simulink model "virtual_hopper_feedback_simplified"  (R2018b)
settings: Solver=ode4  StartTime=0  StopTime=10  FixedStep=0.0005  RelTol=1e-7  AbsTol=1e-9  EnableMultiTasking=on
settings Model: Creator=Laksh  LastModifiedBy=Ko
settings SolverCC: AutoScaleAbsTol=off  MaxConsecutiveMinStep=10  AlgebraicLoopSolver=LineSearch
settings DataIOCC: SaveFormat=StructureWithTime  SignalLogging=off  ReturnWorkspaceOutputs=on
settings OptimizationCC: LifeSpan=inf
settings DebuggingCC: ReadBeforeWriteMsg=DisableAll  WriteAfterWriteMsg=DisableAll  WriteAfterReadMsg=DisableAll  AlgebraicLoopMsg=none  MultiTaskDSMMsg=none  SFUnexpectedBacktrackingDiag=warning  SFNoUnconditionalDefaultTransitionDiag=warning  SFExecutionAtInitializationDiag=none
settings ModelReferenceCC: UpdateModelReferenceTargets=IfOutOfDate  ModelReferenceMinAlgLoopOccurrences=on
settings SFSimCC: SFSimEcho=off  SimUseLocalCustomCode=off
settings RTWCC: RTWUseLocalCustomCode=off
settings CodeAppCC: StateflowObjectComments=on
settings GRTTargetCC: TargetLangStandard=C89/C90 (ANSI)  GeneratePreprocessorConditionals=Disable all
settings ConfigComp: CovMetricSettings=dw  CovHtmlReporting=on  CovSaveCumulativeToWorkspaceVar=on  CovSaveSingleToWorkspaceVar=on  CovExternalEMLEnable=off

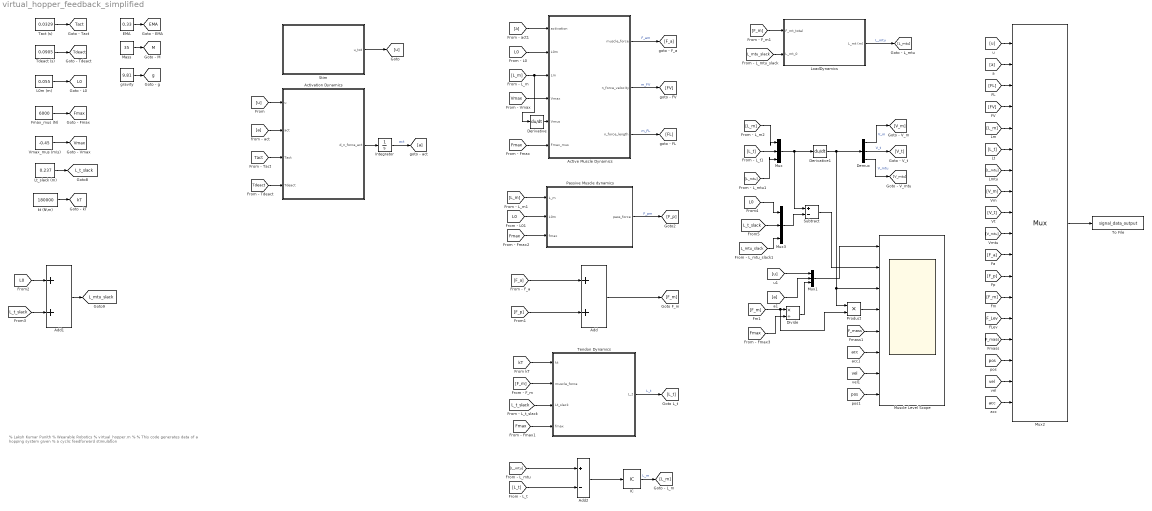
== system virtual_hopper_feedback_simplified ==
  note: % Laksh Kumar Punith
      | % Wearable Robotics
      | % virtual_hopper.m
      | %
      | % This code generates data of a hopping system given
      | % a cyclic feedforward stimulation
  Activation Dynamics : MATLAB Function  TreatAsAtomicUnit=on
  Active Muscle Dynamics : MATLAB Function
  Add : Sum
  Add1 : Sum
  Add2 : Sum  Inputs=+-
  Demux : Demux  Outputs=3
  Derivative : Derivative
  Derivative1 : Derivative
  Divide : Product  Inputs=*/
  EMA : Constant  Value=0.33
  Fmax_mus (N) : Constant  Value=6000
  IC : InitialCondition  Value=0.05
  Integrator : Integrator
  L0m (m) : Constant  Value=0.055
  LoadDynamics : Subsystem
  Lt_slack (m) : Constant  Value=0.237
  Mass : Constant  Value=35
  Muscle Level Scope : Scope  NumInputPorts=8
  Mux : Mux  Inputs=3
  Mux1 : Mux  Inputs=3
  Mux2 : Mux  Inputs=18
      settings: DisplayOption=signals
  Mux3 : Mux  Inputs=3
  Passive Muscle dynamics : MATLAB Function
  Product : Product
  Stim : Subsystem
  Subtract : Sum  Inputs=+-
  Tact (s) : Constant  Value=0.0329  VectorParams1D=off
  Tdeact (s) : Constant  Value=0.0905
  Tendon Dynamics : MATLAB Function
  To File : ToFile  Filename=signal_data_output  MatrixName=data  SaveFormat=Timeseries
  Vmax_mus (m\s) : Constant  Value=-0.45
  gravity : Constant  Value=9.81
  kt (N\m) : Constant  Value=180000
  tag scope: EMA=global, Fmax=global, L0=global, L_mtu_slack=global, L_t_slack=global, M=global, Tact=global, Tdeact=global, Vmax=global, g=global, kT=global
  wires:
  Activation Dynamics/1(d_n_force_act) -> Integrator/1
  Mux2/1 -> To File/1
  [u] -> Activation Dynamics/1(u)
  Integrator/1 -> [a]  "act"
  [a] -> Activation Dynamics/2(act)
  [a] -> Active Muscle Dynamics/1(activation)
  Active Muscle Dynamics/1(muscle_force) -> [F_a]  "F_am"
  Active Muscle Dynamics/3(n_force_length) -> [FL]  "m_FL"
  Active Muscle Dynamics/2(n_force_velocity) -> [FV]  "m_FV"
  Passive Muscle dynamics/1(pass_force) -> [F_p]  "F_pm"
  Tact (s)/1 -> [Tact]
  Tdeact (s)/1 -> [Tdeact]
  L0m (m)/1 -> [L0]
  Fmax_mus (N)/1 -> [Fmax]
  Vmax_mus (m\s)/1 -> [Vmax]
  Lt_slack (m)/1 -> [L_t_slack]
  [L_t_slack] -> Add1/2
  Add1/1 -> [L_mtu_slack]
  [L0] -> Add1/1
  [L0] -> Active Muscle Dynamics/2(L0m)
  [Vmax] -> Active Muscle Dynamics/4(Vmax)
  [Fmax] -> Active Muscle Dynamics/6(Fmax_mus)
  [L0] -> Passive Muscle dynamics/2(L0m)
  [Fmax] -> Passive Muscle dynamics/3(fmax)
  [L_t_slack] -> Tendon Dynamics/3(Lt_slack)
  [Fmax] -> Tendon Dynamics/4(fmax)
  kt (N\m)/1 -> [kT]
  [kT] -> Tendon Dynamics/1(kt)
  [Tact] -> Activation Dynamics/3(Tact)
  [Tdeact] -> Activation Dynamics/4(Tdeact)
  LoadDynamics/1(L_mt (m)) -> [L_mtu]  "L_mtu"
  Add2/1 -> IC/1
  IC/1 -> [L_m]  "L_m"
  [L_mtu_slack] -> LoadDynamics/2(L_mt_0)
  [F_m] -> LoadDynamics/1(F_mt_total)
  Mass/1 -> [M]
  EMA/1 -> [EMA]
  gravity/1 -> [g]
  [L_t] -> Mux/2
  Mux/1 -> Subtract/1, Derivative1/1
  [L_m] -> Mux/1
  [L_mtu] -> Mux/3
  Derivative1/1 -> Product/1, Muscle Level Scope/3, Demux/1
  Demux/1 -> [V_m]  "V_m"
  Demux/2 -> [V_t]  "V_t"
  Demux/3 -> [V_mtu]  "V_mtu"
  [u] -> Mux2/1
  [a] -> Mux2/2
  [FL] -> Mux2/3
  [FV] -> Mux2/4
  [L_m] -> Mux2/5
  [L_t] -> Mux2/6
  [L_mtu] -> Mux2/7
  [V_m] -> Mux2/8
  [V_t] -> Mux2/9
  [V_mtu] -> Mux2/10
  [F_a] -> Mux2/11
  [F_p] -> Mux2/12
  [F_m] -> Mux2/13
  [F_Lev] -> Mux2/14
  [F_mass] -> Mux2/15
  [pos] -> Mux2/16
  [vel] -> Mux2/17
  [acc] -> Mux2/18
  Add/1 -> [F_m]
  Tendon Dynamics/1(L_t) -> [L_t]  "L_t"
  Derivative/1 -> Active Muscle Dynamics/5(Vmus)
  [L_m] -> Passive Muscle dynamics/1(L_m)
  [L_m] -> Derivative/1, Active Muscle Dynamics/3(Lm)
  [F_a] -> Add/1
  [F_p] -> Add/2
  [F_m] -> Tendon Dynamics/2(muscle_force)
  [L_mtu] -> Add2/1
  [L_t] -> Add2/2
  [u] -> Mux1/1
  [a] -> Mux1/2
  Mux1/1 -> Muscle Level Scope/1
  [L0] -> Mux3/1
  [L_t_slack] -> Mux3/2
  [L_mtu_slack] -> Mux3/3
  Mux3/1 -> Subtract/2
  Subtract/1 -> Muscle Level Scope/2
  [F_m] -> Product/2, Divide/1
  [Fmax] -> Divide/2
  Divide/1 -> Mux1/3
  Product/1 -> Muscle Level Scope/4
  [acc] -> Muscle Level Scope/6
  [vel] -> Muscle Level Scope/7
  [pos] -> Muscle Level Scope/8
  [F_mass] -> Muscle Level Scope/5
  Stim/1(u_tot) -> [u]

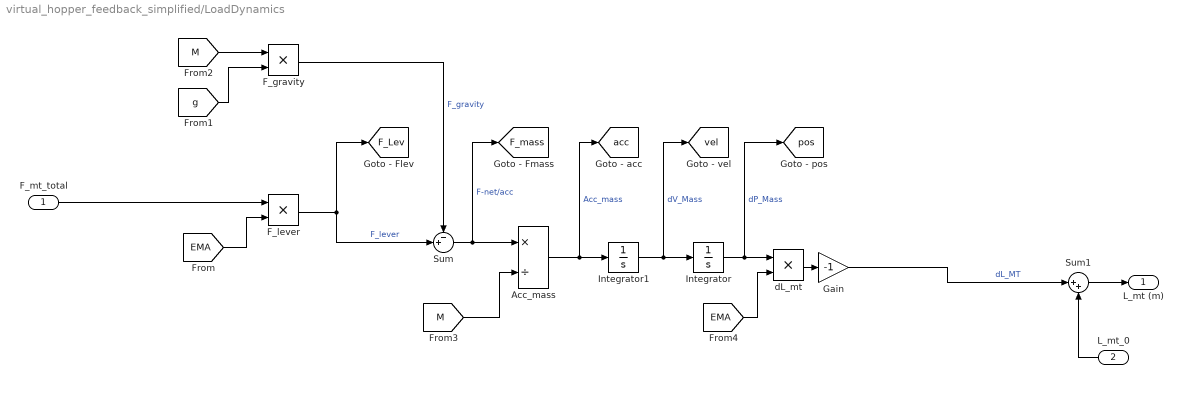
== system virtual_hopper_feedback_simplified/LoadDynamics ==
  F_mt_total : Inport
  L_mt_0 : Inport  Port=2
  Acc_mass : Product  Inputs=*/
  F_gravity : Product  RndMeth=Zero
  F_lever : Product  RndMeth=Zero
  Gain : Gain  Gain=-1
  Integrator : Integrator  InitialCondition=0.05
  Integrator1 : Integrator
  Sum : Sum  Inputs=-+|
  Sum1 : Sum  Inputs=|++
  dL_mt : Product  RndMeth=Zero
  L_mt (m) : Outport
  tag scope: F_Lev=global, F_mass=global, acc=global, pos=global, vel=global
  wires:
  Integrator1/1 -> [vel], Integrator/1  "dV_Mass"
  Sum1/1 -> L_mt (m)/1
  L_mt_0/1 -> Sum1/2
  Acc_mass/1 -> [acc], Integrator1/1  "Acc_mass"
  Sum/1 -> [F_mass], Acc_mass/1  "F-net/acc"
  F_mt_total/1 -> F_lever/1
  Gain/1 -> Sum1/1  "dL_MT"
  dL_mt/1 -> Gain/1
  F_lever/1 -> Sum/2, [F_Lev]  "F_lever"
  [M] -> F_gravity/1
  [g] -> F_gravity/2
  [EMA] -> F_lever/2
  Integrator/1 -> [pos], dL_mt/1  "dP_Mass"
  [M] -> Acc_mass/2
  F_gravity/1 -> Sum/1  "F_gravity"
  [EMA] -> dL_mt/2

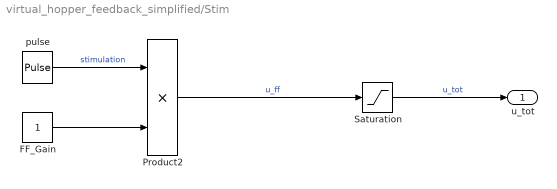
== system virtual_hopper_feedback_simplified/Stim ==
  FF_Gain : Constant
  Product2 : Product
  Saturation : Saturate  UpperLimit=1  LowerLimit=0
  pulse : DiscretePulseGenerator  PulseType=Time based  Period=0.4  PulseWidth=10  PhaseDelay=0.1
  u_tot : Outport
  wires:
  pulse/1 -> Product2/1  "stimulation"
  FF_Gain/1 -> Product2/2
  Product2/1 -> Saturation/1  "u_ff"
  Saturation/1 -> u_tot/1  "u_tot"

== matlab function virtual_hopper_feedback_simplified/Active Muscle Dynamics ==
  data: activation input; L0m input; Lm input; Vmax input; Vmus input; Fmax_mus input; muscle_force output; n_force_velocity output; n_force_length output
function [muscle_force, n_force_velocity, n_force_length]  =...
    muscle_dynamics(activation,L0m,Lm,Vmax,Vmus,Fmax_mus)
%#codegen

    %Hill Type Muscle F-V relationship.  Returns a normalized force-velocity value
    if (Vmus<Vmax)
        n_force_velocity=0;
    else
        if (Vmus >= Vmax && Vmus < 0)
            n_force_velocity = ((1-(Vmus/Vmax))/(1+(Vmus/0.17/Vmax)));
        else
            n_force_velocity =(1.8-0.8*((1+(Vmus/Vmax))/(1-7.56*Vmus/0.17/Vmax)));
        end
    end
    
    %Active muscle F-L relationships.  Returns a normalized F-L value

    a = 3.1108;
    b = .8698;
    s = .3914;

    if Lm < 0
        Lm = 0;
    end

    n_force_length = exp(-(abs(((Lm/L0m)^b-1)/s))^a);

    %Total active force of muscle based on normalized F-V and F-L relationships
    muscle_force = Fmax_mus* activation * n_force_velocity * n_force_length;
end

== matlab function virtual_hopper_feedback_simplified/Tendon Dynamics ==
  data: kt input; L_t output; muscle_force input; Lt_slack input; fmax input
function L_t = L_tendon(kt,muscle_force,Lt_slack,fmax)
%#codegen
%Lichtwark, G.A. and Wilson, A.M., 2008. Journal of theoretical biology, 252(4), pp.662-673.
%Total tendon length
dL_t = (muscle_force + (fmax*log((-9*exp(-(20*muscle_force)/fmax)) + 10))/20)/kt;
L_t = dL_t + Lt_slack ;

end

== matlab function virtual_hopper_feedback_simplified/Activation Dynamics ==
  data: u input; d_n_force_act output; act input; Tact input; Tdeact input
function d_n_force_act = d_n_force_act(u,act,Tact,Tdeact)
%#codegen    
%Rate of change of activation
%Equation is taken from Zajac (1989) Eq. 1
    B=Tact/Tdeact;
    d_n_force_act= u/Tact - (1/Tact*(B+(1-B)*u))*act;
end

== matlab function virtual_hopper_feedback_simplified/Passive Muscle dynamics ==
  data: pass_force output; L_m input; L0m input; fmax input
function pass_force = pmuscle_dynamics(L_m, L0m,fmax)
%#codegen
%passive CE F_L taken from Rubenson et. al.

%Passive muscle force
A = 2.38*10^(-2);
b = 5.31;

if L_m > 0    
    pass_force= fmax*A*exp(b*((L_m/L0m)-1));
else
    pass_force=0;
end


end
